simulink model "Part3"  (R2018a)
settings: Solver=VariableStepAuto  StartTime=0.0  StopTime=2  RelTol=1e-3
libraries: simulink x1
settings Model: Creator=menonpr7  LastModifiedBy=menonpr7

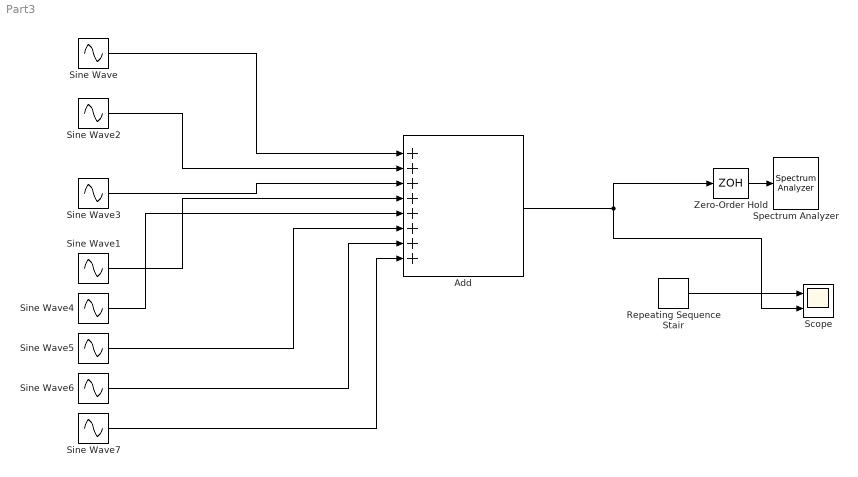
== system Part3 ==
  Add : Sum  Inputs=++++++++
  Repeating Sequence Stair : simulink/Sources/Repeating Sequence Stair  OutValues=[1 -1]  tsamp=1/64  OutMin=[]  OutMax=[]  OutDataTypeStr=double  OutputDataTypeScalingMode=double  OutDataType=fixdt(0,8)  ConRadixGroup=Best Precision: Vector-wise  OutScaling=2^-12
  Scope : Scope  NumInputPorts=2
  Sine Wave : Sin  Amplitude=4/(7*pi)  Frequency=14*32*pi  SampleTime=0
  Sine Wave1 : Sin  Amplitude=4/pi  Frequency=64*pi  SampleTime=0
  Sine Wave2 : Sin  Amplitude=4/(5*pi)  Frequency=10*32*pi  SampleTime=0
  Sine Wave3 : Sin  Amplitude=4/(3*pi)  Frequency=192*pi  SampleTime=0
  Sine Wave4 : Sin  Amplitude=4/(9*pi)  Frequency=18*32*pi  SampleTime=0
  Sine Wave5 : Sin  Amplitude=4/(11*pi)  Frequency=22*32*pi  SampleTime=0
  Sine Wave6 : Sin  Amplitude=4/(13*pi)  Frequency=26*32*pi  SampleTime=0
  Sine Wave7 : Sin  Amplitude=4/(15*pi)  Frequency=30*32*pi  SampleTime=0
  Spectrum Analyzer : SpectrumAnalyzer
  Zero-Order Hold : ZeroOrderHold  SampleTime=2^(-10)
  wires:
  Zero-Order Hold/1 -> Spectrum Analyzer/1
  Repeating Sequence Stair/1 -> Scope/1
  Sine Wave/1 -> Add/1
  Sine Wave2/1 -> Add/2
  Sine Wave3/1 -> Add/3
  Sine Wave1/1 -> Add/4
  Add/1 -> Zero-Order Hold/1, Scope/2
  Sine Wave4/1 -> Add/5
  Sine Wave5/1 -> Add/6
  Sine Wave6/1 -> Add/7
  Sine Wave7/1 -> Add/8
